simulink model "Beobachter"  (R2021b)
settings: Solver=ode8  StartTime=0.0  StopTime=10.0  RelTol=1e-3
model workspace (MAT data in the model file):
  A = Simulink.Parameter
  A.Value = [0  1; 0  0]
  A.DataType = 'auto'
  A.Complexity = 'real'
  A.Dimensions = [2 2]
  B = Simulink.Parameter
  B.Value = [0; 7.007]
  B.DataType = 'auto'
  B.Complexity = 'real'
  B.Dimensions = [2 1]
  C = Simulink.Parameter
  C.Value = [1 0]
  C.DataType = 'auto'
  C.Complexity = 'real'
  C.Dimensions = [1 2]
values from neighbouring files (symbols this model uses):
  K = acker(A,B,p)    [prelude.m]
  L = [[L_T(1,1)];[L_T(1,2)]]    [prelude.m]
settings Model: Creator=Hoorsana  LastModifiedBy=Hoorsana
settings SolverCC: AlgebraicLoopSolver=TrustRegion

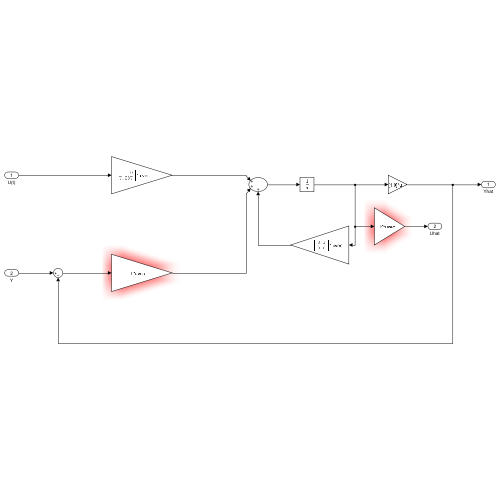
[thumbnail: Simulink's stored preview of the top-level diagram]
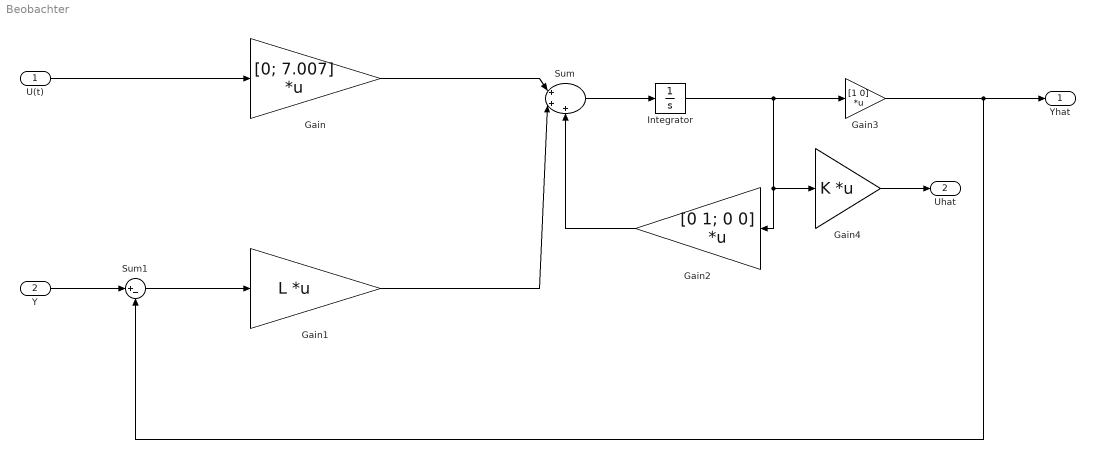
== system Beobachter ==
  U(t) : Inport
  Y : Inport  Port=2
  Gain : Gain  Gain=[0; 7.007]  Multiplication=Matrix(K*u) (u vector)
  Gain1 : Gain  Gain=L  Multiplication=Matrix(K*u) (u vector)
  Gain2 : Gain  Gain=[0 1; 0 0]  Multiplication=Matrix(K*u) (u vector)
  Gain3 : Gain  Gain=[1 0]  Multiplication=Matrix(K*u)
  Gain4 : Gain  Gain=K  Multiplication=Matrix(K*u) (u vector)
  Integrator : Integrator
  Sum : Sum  Inputs=|+++
  Sum1 : Sum  Inputs=|+-
  Yhat : Outport
  Uhat : Outport  Port=2  VectorParamsAs1DForOutWhenUnconnected=off
  wires:
  Sum1/1 -> Gain1/1
  Gain1/1 -> Sum/2
  Integrator/1 -> Gain2/1, Gain4/1, Gain3/1
  Gain2/1 -> Sum/3
  Sum/1 -> Integrator/1
  Gain4/1 -> Uhat/1
  Gain/1 -> Sum/1
  Gain3/1 -> Sum1/2, Yhat/1
  Y/1 -> Sum1/1
  U(t)/1 -> Gain/1
